simulink model "heli_master"  (R2018b)
settings: Solver=ode1  StartTime=0.0  StopTime=8  FixedStep=0.002  RelTol=1e-3  EnableMultiTasking=on
PostLoadFcn:
  | if variant_hil
  |     qc_set_target_type(getConfigSet(bdroot, 'QUARC Default Target Configuration'));
  | end
values from neighbouring files (symbols this model uses):
  lamb = block.ContStates.Data(3)    [BetterSimulation.m]    (also in FeedbackLinearization.m = x(3); dyn_ext_eps_meas.mat = [0 0 0 0 0 0 0 0 0 0 0 0 ... (30000 elements, 6000x5)]; e_-10_10_l_0_120_t_10.mat = [0 3.40359280049e-12 1.08295188827e-10 8.177826625e-10 3.426; e_-10_10_l_0_120_t_20.mat = [0 1.06295178385e-13 3.38915391498e-12 2.56636695446e-11 1.0)
  phi = block.ContStates.Data(1)    [BetterSimulation.m]    (also in FeedbackLinearization.m = x(1); dyn_ext_eps_meas.mat = [0 0 0 0 0 0 0 0 0 0 0 0 ... (18000 elements, 6000x3)]; e_-10_10_l_0_120_t_10.mat = [3.57789727367e-14 3.32260230971e-07 2.63920782562e-06 8.843; e_-10_10_l_0_120_t_20.mat = [3.52494450884e-15 1.04005854531e-08 8.29611824462e-08 2.791)
  vb = block.InputPort(2).Data    [BetterSimulation.m]    (also in analyze_eps_meas.m = [log_neg.signals(2).values; log_pos.signals(2).values]; dyn_ext_eps_meas.mat = [2.46662433384 2.46662437608 2.46662467016 2.46662546356 2.4; e_-10_10_l_0_120_t_10.mat = [3.03305943788 3.0306076999 3.02819113358 3.02581096907 3.02; e_-10_10_l_0_120_t_20.mat = [3.03305943788 3.0329822422 3.03290486178 3.03282733913 3.03)
  vf = block.InputPort(1).Data    [BetterSimulation.m]    (also in analyze_eps_meas.m = [log_neg.signals(1).values; log_pos.signals(1).values]; dyn_ext_eps_meas.mat = [2.46662433384 2.46662437608 2.46662467016 2.46662546356 2.4; e_-10_10_l_0_120_t_10.mat = [3.03305943788 3.03551133878 3.03792903521 3.04031223633 3.0; e_-10_10_l_0_120_t_20.mat = [3.03305943788 3.03313663866 3.03321405463 3.03329167331 3.0)
undefined symbols (not defined in the file or in its folder): HIL, qc_get_step_size
libraries: quarc_library x3, simulink_extras x3
settings Model: ExtModeTrigDuration=5000  Creator=Rchan  LastModifiedBy=Robert
settings SolverCC: PositivePriorityOrder=on
settings DataIOCC: LimitDataPoints=on  SaveFormat=Array  SignalLoggingSaveFormat=ModelDataLogs
settings OptimizationCC: ExpressionDepthLimit=2147483647  InitFltsAndDblsToZero=on  LifeSpan=inf
settings DebuggingCC: SaveWithParameterizedLinksMsg=none  UnderspecifiedInitializationDetection=Classic  MergeDetectMultiDrivingBlocksExec=none  SolverPrmCheckMsg=warning  MultiTaskDSMMsg=warning  MultiTaskCondExecSysMsg=none  FcnCallInpInsideContextMsg=warning  StateNameClashWarn=warning  SFUnexpectedBacktrackingDiag=warning  SFNoUnconditionalDefaultTransitionDiag=warning  SFExecutionAtInitializationDiag=none
settings HardwareCC: ProdBitPerPointer=32  ProdBitPerSizeT=32  ProdBitPerPtrDiffT=32  ProdLargestAtomicFloat=None  ProdIntDivRoundTo=Undefined  ProdEndianess=Unspecified  ProdWordSize=32  ProdHWDeviceType=32-bit Generic
settings ModelReferenceCC: PropagateSignalLabelsOutOfModel=off
settings SFSimCC: SimUseLocalCustomCode=off
settings RTWCC: SystemTargetFile=quarc_win64.tlc  TemplateMakefile=quarc_default_tmf  Description=QUARC Win64 Target  RTWUseLocalCustomCode=off
settings CodeAppCC: StateflowObjectComments=on
settings STFCustomTargetCC: TargetPreCompLibLocation=D:\PROGRA~3\QUARC\lib\2014a\win64\release  ConcurrentExecutionCompliant=on  GeneratePreprocessorConditionals=Disable all  CPPClassGenCompliant=on  GRTInterface=on  SystemTargetFile=quarc_win64.tlc
settings GRTTargetCC: TargetPreCompLibLocation=D:\PROGRA~3\QUARC\lib\2014a\win64\release  TargetLangStandard=C89/C90 (ANSI)  ParMdlRefBuildCompliant=off  CompOptLevelCompliant=off  GeneratePreprocessorConditionals=Disable all  CombineOutputUpdateFcns=off  MatFileLogging=off  GRTInterface=on  UseToolchainInfoCompliant=off  ExtMode=on  ExtModeMexFile=quarc_comm
settings ConfigComp: CovMetricSettings=dw  CovHtmlReporting=on  CovSaveCumulativeToWorkspaceVar=on  CovSaveSingleToWorkspaceVar=on  CovExternalEMLEnable=off  CovSFcnEnable=off

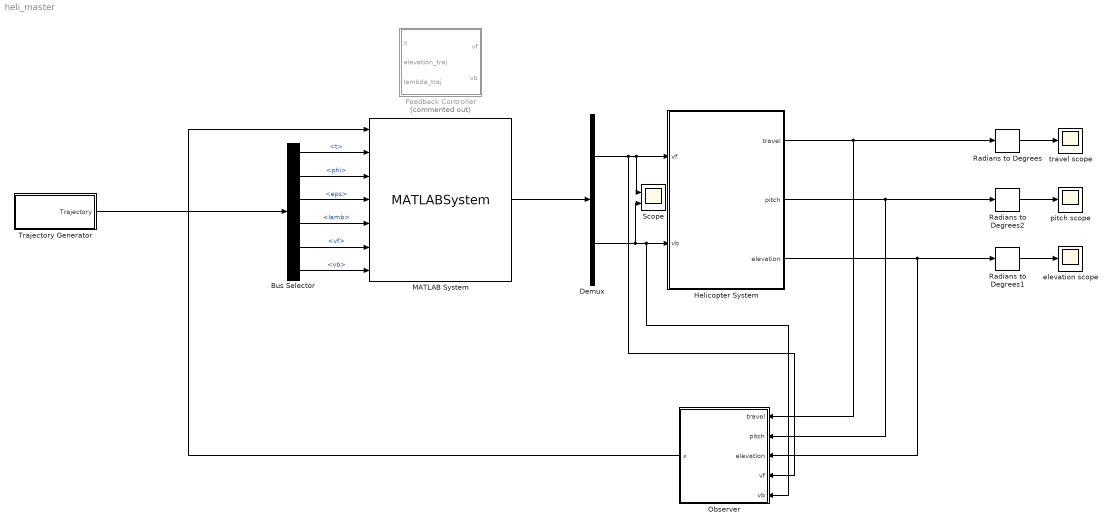
== system heli_master ==
  Bus Selector : BusSelector  OutputSignals=t,phi,eps,lamb,vf,vb
  Demux : Demux  Outputs=2
  Feedback Controller : Subsystem  Commented=on
  Helicopter System : Subsystem  VariantControlMode=Label  Variant=on  LabelModeActiveChoice=var_sim
  MATLAB System : MATLABSystem  System=CascadePid  elevation_pid_gains=[ 10, 2, 5 ]  travel_pitch_pid_gains=[ 1.5, 0.1, 1.5 ]  pitch_vd_pid_gains=[ 20, 0, 2.3 ]  SimulateUsing=Code generation
      mask Type: CascadePid
      mask Display:
      | disp('CascadePid');
      | port_label('input',1,'State');
      | port_label('input',2,'Traj Time');
      | port_label('input',3,'Traj Phi');
      | port_label('input',4,'Traj Eps');
      | port_label('input',5,'Traj Lamb');
      | port_label('input',6,'Traj Vf');
      | port_label('input',7,'Traj Vb');
      | port_label('output',1,'Control');
  Observer : Subsystem
  Radians to Degrees : simulink_extras/Transformations/Radians to Degrees
  Radians to Degrees1 : simulink_extras/Transformations/Radians to Degrees
  Radians to Degrees2 : simulink_extras/Transformations/Radians to Degrees
  Scope : Scope  NumInputPorts=2
  Trajectory Generator : Subsystem
  elevation scope : Scope
  pitch scope : Scope
  travel scope : Scope
  wires:
  Helicopter System/1(travel) -> Observer/1(travel), Radians to Degrees/1
  Helicopter System/3(elevation) -> Observer/3(elevation), Radians to Degrees1/1
  Helicopter System/2(pitch) -> Observer/2(pitch), Radians to Degrees2/1
  Radians to Degrees/1 -> travel scope/1
  Radians to Degrees2/1 -> pitch scope/1
  Radians to Degrees1/1 -> elevation scope/1
  Demux/2 -> Scope/2, Observer/5(vb), Helicopter System/2(vb)
  Demux/1 -> Observer/4(vf), Scope/1, Helicopter System/1(vf)
  MATLAB System/1 -> Demux/1
  Observer/1(x) -> MATLAB System/1
  Trajectory Generator/1(Trajectory) -> Bus Selector/1
  Bus Selector/1 -> MATLAB System/2  "<t>"
  Bus Selector/2 -> MATLAB System/3  "<phi>"
  Bus Selector/3 -> MATLAB System/4  "<eps>"
  Bus Selector/4 -> MATLAB System/5  "<lamb>"
  Bus Selector/5 -> MATLAB System/6  "<vf>"
  Bus Selector/6 -> MATLAB System/7  "<vb>"

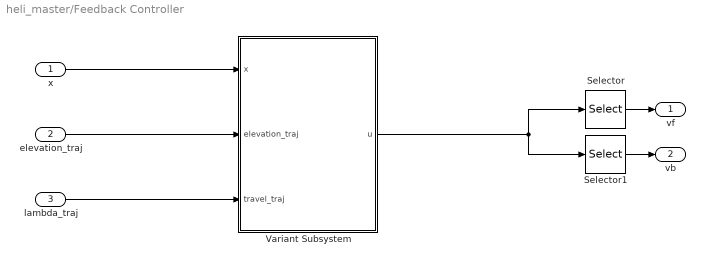
== system heli_master/Feedback Controller ==
  x : Inport
  elevation_traj : Inport  Port=2
  lambda_traj : Inport  Port=3
  Selector : Selector  InputPortWidth=2  IndexOptions=Index vector (dialog)  Indices=1  OutputSizes=1
  Selector1 : Selector  InputPortWidth=2  IndexOptions=Index vector (dialog)  Indices=2  OutputSizes=1
  Variant Subsystem : Subsystem  VariantControlMode=Label  Variant=on  LabelModeActiveChoice=TIME_VARIANT_LQR
  vf : Outport
  vb : Outport  Port=2
  wires:
  Selector/1 -> vf/1
  Selector1/1 -> vb/1
  elevation_traj/1 -> Variant Subsystem/2(elevation_traj)
  x/1 -> Variant Subsystem/1(x)
  lambda_traj/1 -> Variant Subsystem/3(travel_traj)
  Variant Subsystem/1(u) -> Selector/1, Selector1/1

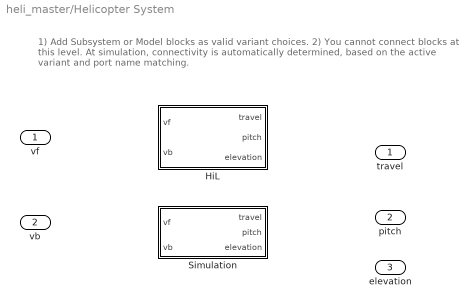
== system heli_master/Helicopter System ==
  note: 1) Add Subsystem or Model blocks as valid variant choices.
      | 2) You cannot connect blocks at this level. At simulation, connectivity is automatically
      | determined, based on the active variant and port name matching.
  vf : Inport
  vb : Inport  Port=2
  HiL : Subsystem  VariantControl=var_hil
  Simulation : Subsystem  VariantControl=var_sim
  travel : Outport
  pitch : Outport  Port=2
  elevation : Outport  Port=3

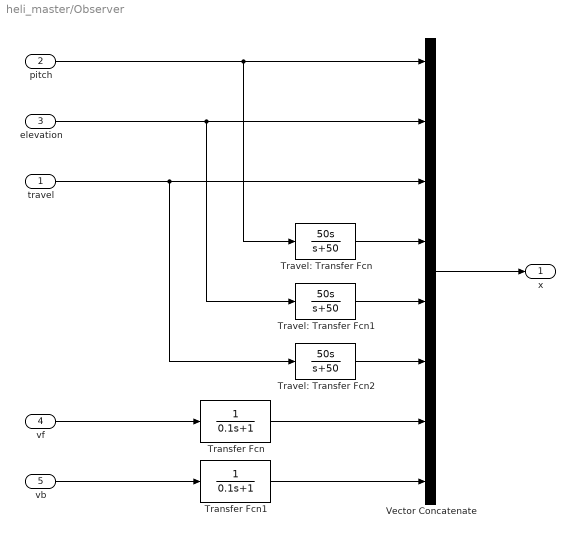
== system heli_master/Observer ==
  travel : Inport
  pitch : Inport  Port=2
  elevation : Inport  Port=3
  vf : Inport  Port=4
  vb : Inport  Port=5
  Transfer Fcn : TransferFcn  Denominator=[0.1 1]
  Transfer Fcn1 : TransferFcn  Denominator=[0.1 1]
  Travel: Transfer Fcn : TransferFcn  Numerator=[50 0]  Denominator=[1 50]
  Travel: Transfer Fcn1 : TransferFcn  Numerator=[50 0]  Denominator=[1 50]
  Travel: Transfer Fcn2 : TransferFcn  Numerator=[50 0]  Denominator=[1 50]
  Vector Concatenate : Concatenate  NumInputs=8
  x : Outport
  wires:
  pitch/1 -> Travel: Transfer Fcn/1, Vector Concatenate/1
  elevation/1 -> Vector Concatenate/2, Travel: Transfer Fcn1/1
  travel/1 -> Vector Concatenate/3, Travel: Transfer Fcn2/1
  Vector Concatenate/1 -> x/1
  Travel: Transfer Fcn/1 -> Vector Concatenate/4
  Travel: Transfer Fcn1/1 -> Vector Concatenate/5
  Travel: Transfer Fcn2/1 -> Vector Concatenate/6
  Transfer Fcn/1 -> Vector Concatenate/7
  vf/1 -> Transfer Fcn/1
  Transfer Fcn1/1 -> Vector Concatenate/8
  vb/1 -> Transfer Fcn1/1

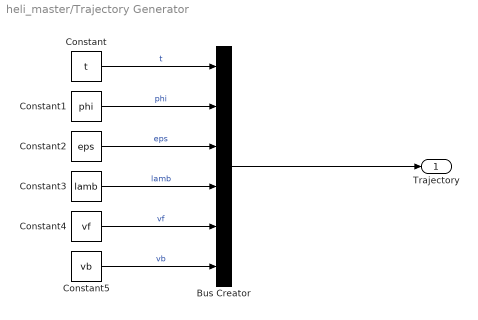
== system heli_master/Trajectory Generator ==
  Bus Creator : BusCreator  Inputs=6
  Constant : Constant  Value=t
  Constant1 : Constant  Value=phi
  Constant2 : Constant  Value=eps
  Constant3 : Constant  Value=lamb
  Constant4 : Constant  Value=vf
  Constant5 : Constant  Value=vb
  Trajectory : Outport
  wires:
  Constant/1 -> Bus Creator/1  "t"
  Constant5/1 -> Bus Creator/6  "vb"
  Constant4/1 -> Bus Creator/5  "vf"
  Constant3/1 -> Bus Creator/4  "lamb"
  Constant2/1 -> Bus Creator/3  "eps"
  Constant1/1 -> Bus Creator/2  "phi"
  Bus Creator/1 -> Trajectory/1

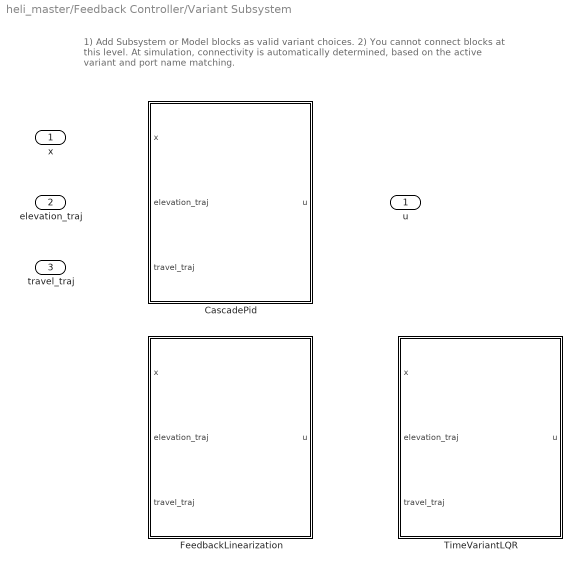
== system heli_master/Feedback Controller/Variant Subsystem ==
  note: 1) Add Subsystem or Model blocks as valid variant choices.
      | 2) You cannot connect blocks at this level. At simulation, connectivity is automatically
      | determined, based on the active variant and port name matching.
  x : Inport
  elevation_traj : Inport  Port=2
  travel_traj : Inport  Port=3
  CascadePid : Subsystem  VariantControl=CASCADE_PID
  FeedbackLinearization : Subsystem  VariantControl=FEEDBACK_LINEARIZATION
  TimeVariantLQR : Subsystem  VariantControl=TIME_VARIANT_LQR
  u : Outport

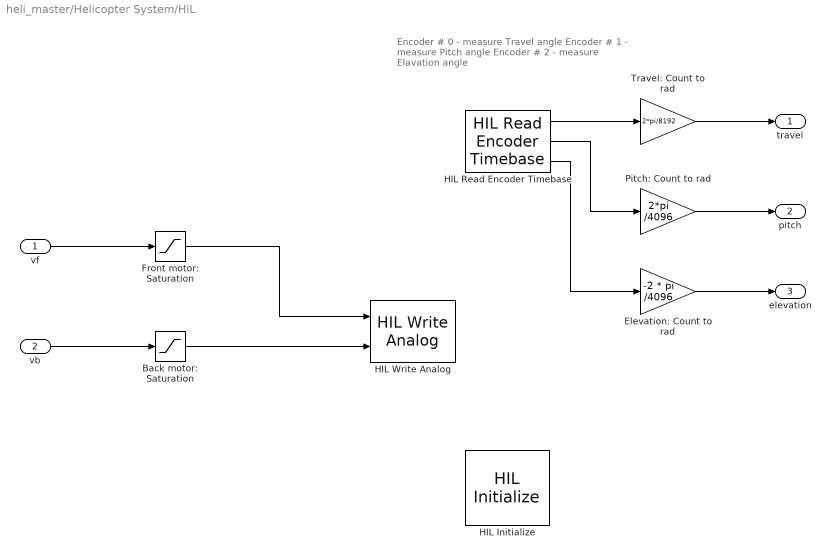
== system heli_master/Helicopter System/HiL ==
  note: Encoder # 0 - measure Travel angle
      | Encoder # 1 - measure Pitch angle
      | Encoder # 2 - measure Elavation angle
  vf : Inport
  vb : Inport  Port=2
  Back motor: Saturation : Saturate  UpperLimit=5  LowerLimit=-5
  Elevation: Count to rad : Gain  Gain=-2 * pi /4096
  Front motor: Saturation : Saturate  UpperLimit=5  LowerLimit=-5
  HIL Initialize : quarc_library/Data Acquisition/Generic/Configuration/HIL Initialize  Priority=-99  object_name=HIL-1  board_type=q8_usb  board_number=0  board_options=update_rate=normal;decimation=1  exclusive=off  active=off  hardware_clocks=[0:2]  clock_modes=[]  initial_clock_frequencies=[]  set_clock_params_at_start=off  set_clock_params_at_switch_in=off  set_clock_frequencies_at_start=off  set_clock_frequencies_at_switch_in=off  analog_input_channels=[0:7]  analog_input_maximums=10  analog_input_minimums=-10  set_analog_input_params_at_start=on  set_analog_input_params_at_switch_in=off  analog_output_channels=[0:7]  analog_output_maximums=10  analog_output_minimums=-10  initial_analog_outputs=[0]  final_analog_outputs=[0]  watchdog_analog_outputs=0  set_analog_output_params_at_start=on  set_analog_output_params_at_switch_in=off  set_analog_outputs_at_start=on  set_analog_outputs_at_switch_in=off  set_analog_outputs_at_terminate=on  set_analog_outputs_at_switch_out=off  set_analog_outputs_on_watchdog=off  digital_input_channels=[]  digital_output_channels=[]  digital_output_configuration=[]  initial_digital_outputs=[1]  final_digital_outputs=[1]  watchdog_digital_outputs=[1]  set_digital_output_params_at_start=off  set_digital_output_params_at_switch_in=off  set_digital_outputs_at_start=on  set_digital_outputs_at_switch_in=off  set_digital_outputs_at_terminate=on  set_digital_outputs_at_switch_out=off  set_digital_outputs_on_watchdog=off  encoder_channels=[0:7]  quadrature=[4]  encoder_filter_frequency=[]  initial_encoder_counts=[0]  set_encoder_params_at_start=on  set_encoder_params_at_switch_in=off  set_encoder_counts_at_start=on  set_encoder_counts_at_switch_in=off  pwm_channels=[0:7]  pwm_modes=0  pwm_frequency=99.532799999999995e6/4095  pwm_configuration=[0]  pwm_alignment=[0]  pwm_polarity=[1]  pwm_leading_deadband=[0]  pwm_trailing_deadband=[0]  initial_pwm_outputs=[0]  final_pwm_outputs=[0]  watchdog_pwm_outputs=[0]  set_pwm_params_at_start=on  set_pwm_params_at_switch_in=off  set_pwm_outputs_at_start=on  set_pwm_outputs_at_switch_in=off  set_pwm_outputs_at_terminate=on  set_pwm_outputs_at_switch_out=off  set_pwm_outputs_on_watchdog=off  other_output_channels=[]  initial_other_outputs=[]  final_other_outputs=[]  watchdog_other_outputs=[]  set_other_outputs_at_start=off  set_other_outputs_at_switch_in=off  set_other_outputs_at_terminate=off  set_other_outputs_at_switch_out=off  set_other_outputs_on_watchdog=off
  HIL Read Encoder Timebase : quarc_library/Data Acquisition/Generic/Timebases/HIL Read Encoder Timebase  object_name=HIL-1  clock=0  channels=[0:2]  samples_in_buffer=max(ceil(1/qc_get_step_size), 1)  active=on  vector_output=off  data_type_mode=Inherit via back propagation  data_type=double
  HIL Write Analog : quarc_library/Data Acquisition/Generic/Immediate I//O/HIL Write Analog  object_name=HIL-1  channels=[0:1]  sample_time=-1  active=off  vector_input=off
  Pitch: Count to rad : Gain  Gain=2*pi /4096
  Travel: Count to rad : Gain  Gain=2*pi/8192
  travel : Outport
  pitch : Outport  Port=2
  elevation : Outport  Port=3
  wires:
  vf/1 -> Front motor: Saturation/1
  vb/1 -> Back motor: Saturation/1
  Back motor: Saturation/1 -> HIL Write Analog/2
  HIL Read Encoder Timebase/2 -> Pitch: Count to rad/1
  HIL Read Encoder Timebase/1 -> Travel: Count to rad/1
  Front motor: Saturation/1 -> HIL Write Analog/1
  HIL Read Encoder Timebase/3 -> Elevation: Count to rad/1
  Travel: Count to rad/1 -> travel/1
  Pitch: Count to rad/1 -> pitch/1
  Elevation: Count to rad/1 -> elevation/1

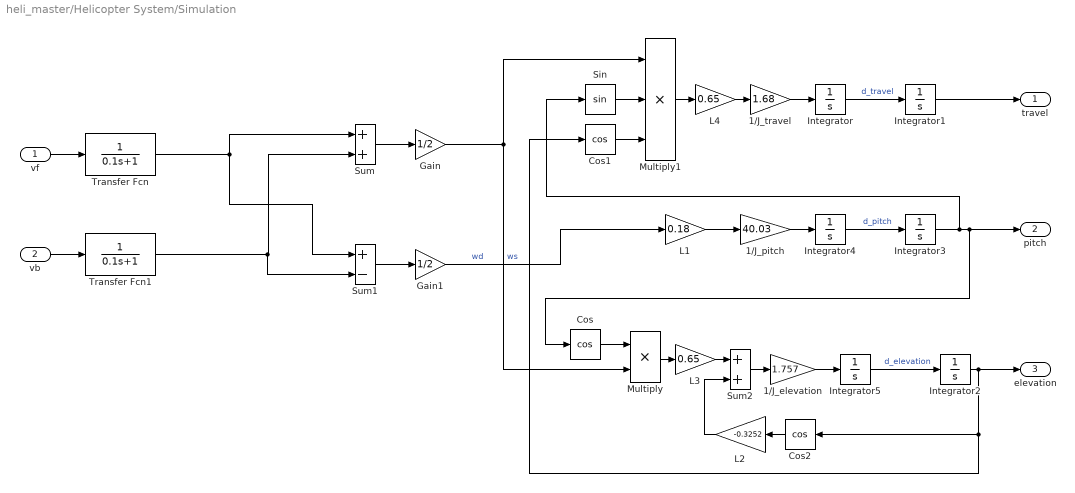
== system heli_master/Helicopter System/Simulation ==
  vf : Inport
  vb : Inport  Port=2
  1/J_elevation : Gain  Gain=1.757
  1/J_pitch : Gain  Gain=40.03
  1/J_travel : Gain  Gain=1.68
  Cos : Trigonometry  Operator=cos
  Cos1 : Trigonometry  Operator=cos
  Cos2 : Trigonometry  Operator=cos
  Gain : Gain  Gain=1/2
  Gain1 : Gain  Gain=1/2
  Integrator : Integrator
  Integrator1 : Integrator  LimitOutput=on  UpperSaturationLimit=2.1  LowerSaturationLimit=-2.1
  Integrator2 : Integrator  LimitOutput=on  UpperSaturationLimit=1.22  LowerSaturationLimit=-1.22
  Integrator3 : Integrator  LimitOutput=on  UpperSaturationLimit=1.4  LowerSaturationLimit=-1.4
  Integrator4 : Integrator
  Integrator5 : Integrator
  L1 : Gain  Gain=0.18
  L2 : Gain  Gain=-0.3252
  L3 : Gain  Gain=0.65
  L4 : Gain  Gain=0.65
  Multiply : Product
  Multiply1 : Product  Inputs=3
  Sin : Trigonometry
  Sum : Sum
  Sum1 : Sum  Inputs=+-
  Sum2 : Sum
  Transfer Fcn : TransferFcn  Denominator=[0.1 1]
  Transfer Fcn1 : TransferFcn  Denominator=[0.1 1]
  travel : Outport
  pitch : Outport  Port=2
  elevation : Outport  Port=3
  wires:
  Integrator/1 -> Integrator1/1  "d_travel"
  Integrator1/1 -> travel/1
  Integrator3/1 -> Sin/1, Cos/1, pitch/1
  Integrator4/1 -> Integrator3/1  "d_pitch"
  Integrator2/1 -> Cos2/1, Cos1/1, elevation/1
  Integrator5/1 -> Integrator2/1  "d_elevation"
  Sum/1 -> Gain/1
  Sum1/1 -> Gain1/1
  1/J_pitch/1 -> Integrator4/1
  L1/1 -> 1/J_pitch/1
  Gain1/1 -> L1/1  "wd"
  Cos/1 -> Multiply/1
  Gain/1 -> Multiply1/1, Multiply/2  "ws"
  1/J_elevation/1 -> Integrator5/1
  1/J_travel/1 -> Integrator/1
  Multiply/1 -> L3/1
  Multiply1/1 -> L4/1
  L4/1 -> 1/J_travel/1
  Sin/1 -> Multiply1/2
  Cos1/1 -> Multiply1/3
  Sum2/1 -> 1/J_elevation/1
  L3/1 -> Sum2/1
  L2/1 -> Sum2/2
  Cos2/1 -> L2/1
  vf/1 -> Transfer Fcn/1
  vb/1 -> Transfer Fcn1/1
  Transfer Fcn/1 -> Sum1/1, Sum/1
  Transfer Fcn1/1 -> Sum1/2, Sum/2

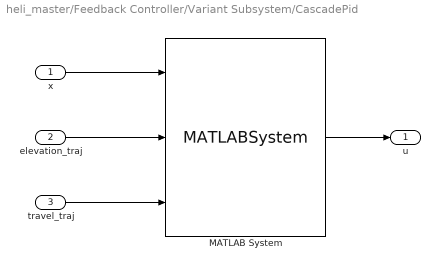
== system heli_master/Feedback Controller/Variant Subsystem/CascadePid ==
  x : Inport
  elevation_traj : Inport  Port=2
  travel_traj : Inport  Port=3
  MATLAB System : MATLABSystem  System=CascadePid  elevation_pid_gains=[ 10, 2, 5 ]  travel_pitch_pid_gains=[ 1.5, 0.1, 1.5 ]  pitch_vd_pid_gains=[ 20, 0, 2.3 ]  SimulateUsing=Code generation
      mask Type: CascadePid
      mask Display:
      | disp('CascadePid');
      | port_label('input',1,'State');
      | port_label('input',2,'Elevation');
      | port_label('input',3,'Travel');
      | port_label('output',1,'Control');
  u : Outport
  wires:
  MATLAB System/1 -> u/1
  x/1 -> MATLAB System/1
  elevation_traj/1 -> MATLAB System/2
  travel_traj/1 -> MATLAB System/3

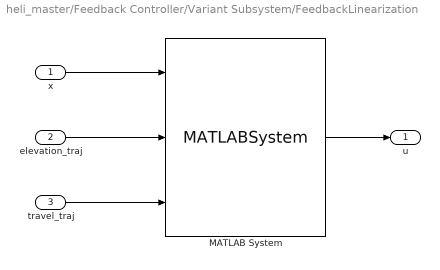
== system heli_master/Feedback Controller/Variant Subsystem/FeedbackLinearization ==
  x : Inport
  elevation_traj : Inport  Port=2
  travel_traj : Inport  Port=3
  MATLAB System : MATLABSystem  System=FeedbackLinearization  friction_centripetal=on  rotor_speed_controller=on  ke=[ 20, 6 ]  kl=[ 1, 0.8 ]  kp=[ 150, 20 ]  k_rotor=[ 5, 0 ]  SimulateUsing=Code generation
      mask Type: FeedbackLinearization
      mask Display:
      | disp('FeedbackLinearization');
      | port_label('input',1,'State');
      | port_label('input',2,'Elevation');
      | port_label('input',3,'Travel');
      | port_label('output',1,'Control');
  u : Outport
  wires:
  MATLAB System/1 -> u/1
  x/1 -> MATLAB System/1
  elevation_traj/1 -> MATLAB System/2
  travel_traj/1 -> MATLAB System/3

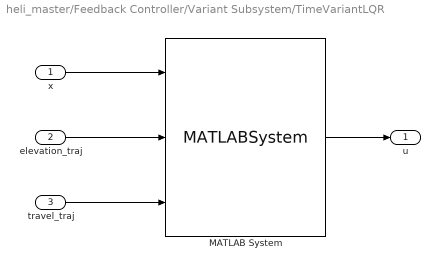
== system heli_master/Feedback Controller/Variant Subsystem/TimeVariantLQR ==
  x : Inport
  elevation_traj : Inport  Port=2
  travel_traj : Inport  Port=3
  MATLAB System : MATLABSystem  System=TimeVariantLQR  Q_diag=[ 2, 10, 4, 0.2, 0.2, 0.1 ]  R_diag=[ 0.1, 0.1 ]  S_diag=[ 1, 1, 1, 0.1, 0.1, 0.1 ]  riccati_step_width=0.1  SimulateUsing=Code generation
      mask Type: TimeVariantLQR
      mask Display:
      | disp('TimeVariantLQR');
      | port_label('input',1,'State');
      | port_label('input',2,'Elevation');
      | port_label('input',3,'Travel');
      | port_label('output',1,'Control');
  u : Outport
  wires:
  MATLAB System/1 -> u/1
  x/1 -> MATLAB System/1
  elevation_traj/1 -> MATLAB System/2
  travel_traj/1 -> MATLAB System/3
